simulink model "AR4FullPositionControl"  (R2026a)
settings: Solver=FixedStepAuto  StopTime=inf  FixedStep=3e-5
PreLoadFcn:
  | load('last_pos.mat');
StopFcn:
  | save('last_pos.mat', 'posJ6', 'posJ5', 'posJ4', 'posJ3', 'posJ2', 'posJ1', 'lastX', 'lastY', 'lastZ');
undefined symbols (not defined in the file): targetColor, targetGo, targetX, targetY, targetZ
libraries: arduinolib x31
(part 3 of 3)

== matlab function AR4FullPositionControl/Subsystem/J1/MATLAB Function1 ==
  data: startNext input; clk input; count output; dt input; rst input; displaySpeed output; dir output; pul output; next output; speedRPM input; positionAngle input; currCount input; accelRPMperSec input; limit output; mode input; homed output
function [count, displaySpeed, dir, pul, next, limit, homed] = J1(startNext, clk, dt, rst, speedRPM, positionAngle, currCount, accelRPMperSec, mode)
% J1 - Joint 1 position/speed controller with S-curve acceleration + HOMING
%
% AR4-MK3 robot. SINGLE-LIMIT joint.
% Limit switch at the most-positive end (+170 deg) = count 0.
% Count increases as the joint moves AWAY from the switch.
%
% MODE (single input):
%   mode = 0  ->  POSITION  : normal operation, drive to positionAngle input
%   mode = 1  ->  INITIALIZE: drive to HOME_TARGET, ignore positionAngle
%   mode = 2  ->  HOMING    : drive toward limit switch, zero count on contact
%
% Typical sequence: 2 (home) -> 1 (go to home angle) -> 0 (position control)
%
% INPUTS
%   startNext, clk, dt, rst, t, speedRPM, positionAngle, currCount,
%   accelRPMperSec, mode  (mode: 0=position, 1=initialize, 2=homing)
% OUTPUTS
%   count, displaySpeed, dir, pul, next, limit, homed
%
%   >>> J1: countsPerDeg=108.78  span=340 deg (-170..170)  maxCount=37500

    persistent currentCount lastClkState lastCount spTimer smoothedSpeed ...
               currentRPM distTraveled totalMoveFrozen lastTarget pulseAccum ...
               homedFlag lastMode;
    persistent chatterAccum chatterDir isStationary;

    % -------------------------------------------------------------------------
    % CONSTANTS  -  per-joint values
    % -------------------------------------------------------------------------
    Ts           = 3e-5;
    PPR          = 1000;
    CPR          = PPR * 4;
    maxCount     = 37500;          % <<< J1
    LIMIT_BUFFER = 50;
    TUNE_C2R     = 0.8;            % <<< J1

    TOTAL_DEG      = 340;          % <<< J1 span: 170-(-170)
    COUNTS_PER_REV = maxCount / TOTAL_DEG * 360;
    GEAR_RATIO     = COUNTS_PER_REV / CPR;
    C2R            = (GEAR_RATIO * CPR) / 60 * TUNE_C2R;

    speedUpdateInterval = 0.2;
    ALPHA               = 0.3;
    MIN_RPM             = 0.5;
    STOP_COUNTS         = 1;

    HOME_RPM    = 3;               % <<< tune: homing speed (RPM)
    HOME_TARGET = 90;               % <<< angle commanded in mode=1 (deg)

    % Single-limit angle->count mapping (anchored at switch)
    J_MIN_DEG    = -170;           % <<< J1
    J_MAX_DEG    =  170;           % <<< J1
    SWITCH_DEG   =  170;           % <<< J1 switch at +170 deg = count 0
    countsPerDeg = maxCount / TOTAL_DEG;

    % -------------------------------------------------------------------------
    % INITIALISATION (first call only)
    % -------------------------------------------------------------------------
    if isempty(currentCount)
        currentCount    = currCount;
        lastCount       = currCount;
        lastClkState    = clk;
        spTimer         = 0;
        smoothedSpeed   = 0;
        currentRPM      = MIN_RPM;
        distTraveled    = 0;
        totalMoveFrozen = 0;
        lastTarget      = -1;
        pulseAccum      = 0;
        homedFlag       = false;
        lastMode        = 0;
        chatterAccum    = 0;
        chatterDir      = 0;
        isStationary    = false;
    end

    limit = false;
    homed = homedFlag;
    dir   = 0;
    pul   = 0;
    next  = false;

    % -------------------------------------------------------------------------
    % 1. ENCODER COUNTING  (stop-triggered freeze)
    %
    % When the joint is stationary (last cycle's absError <= STOP_COUNTS),
    % ALL encoder edges are ignored -- the joint isn't supposed to be moving,
    % so any edge in that state is noise (encoder disk resting on a segment
    % boundary), not real motion. This is a hard freeze, not a filtered
    % accept: no edge can ever nudge currentCount while stationary, which
    % means no per-stop drift, and therefore no drift accumulation across
    % repeated stop events either.
    %
    % The moment a new target actually asks the joint to move (absError
    % grows past STOP_COUNTS, isStationary goes false), counting resumes
    % immediately and every edge is applied normally -- no debounce lag on
    % real motion.
    % -------------------------------------------------------------------------
    if clk ~= lastClkState && clk == 1
        if dt ~= clk
            edgeDir = 1;
        else
            edgeDir = -1;
        end

        if isStationary
            % FULL FREEZE while stationary. Any edge here is, by definition,
            % noise (the joint isn't supposed to be moving), so it's ignored
            % outright rather than "maybe accepted" -- this is what prevents
            % drift from accumulating across repeated stop events. Real
            % counting resumes automatically the moment isStationary goes
            % false (a new target actually asks the joint to move).
            chatterAccum = 0;
            chatterDir   = 0;
        else
            currentCount = currentCount + edgeDir;
            chatterAccum = 0;
            chatterDir   = 0;
        end
    end

    % Reset S-curve state on any mode change (once, on the transition)
    if mode ~= lastMode
        distTraveled    = 0;
        totalMoveFrozen = 0;
        pulseAccum      = 0;
        lastTarget      = -1;
        currentRPM      = MIN_RPM;
        spTimer         = 0;
        smoothedSpeed   = 0;
        chatterAccum    = 0;
        chatterDir      = 0;
    end
    lastMode = mode;

    % =========================================================================
    % MODE 2: HOMING
    % =========================================================================
    if mode == 2
        if rst == 1
            currentCount = 0;
            homedFlag    = true;
        end
        homed = homedFlag;          % limit NOT asserted during homing

        if homedFlag
            currentCount = 0;
            pul          = 0;
            next         = true;
        elseif startNext
            dir        = 0;         % toward switch = decreasing count
            pulseAccum = pulseAccum + HOME_RPM * C2R * Ts;
            if pulseAccum >= 1.0
                pul        = 1;
                pulseAccum = pulseAccum - 1.0;
            end
        end

        count        = currentCount;
        displaySpeed = HOME_RPM;
        lastClkState = clk;
        isStationary = false;
        return;
    end
    % =========================================================================

    % -------------------------------------------------------------------------
    % 2. SPEED DISPLAY
    % -------------------------------------------------------------------------
    spTimer = spTimer + Ts;
    if spTimer >= speedUpdateInterval
        smoothedSpeed = ALPHA * currentRPM + (1 - ALPHA) * smoothedSpeed;
        spTimer       = 0;
    end

    % -------------------------------------------------------------------------
    % 3. TARGET FROM ANGLE
    %    mode 1 (INITIALIZE): command = HOME_TARGET
    %    mode 0 (POSITION)  : command = positionAngle input
    % -------------------------------------------------------------------------
    if mode == 1
        cmdAngle = HOME_TARGET;
    else
        cmdAngle = positionAngle;
    end

    % Clamp to physical range, then map (single-limit, anchored at switch)
    if cmdAngle < J_MIN_DEG, cmdAngle = J_MIN_DEG; end
    if cmdAngle > J_MAX_DEG, cmdAngle = J_MAX_DEG; end
    targetCount = round(abs(SWITCH_DEG - cmdAngle) * countsPerDeg);
    targetCount = max(LIMIT_BUFFER, min(maxCount - LIMIT_BUFFER, targetCount));

    % -------------------------------------------------------------------------
    % 4. DIRECTION
    % -------------------------------------------------------------------------
    countError = targetCount - currentCount;
    absError   = abs(countError);
    if countError >= 0
        dir = 1;
    else
        dir = 0;
    end

    % -------------------------------------------------------------------------
    % 5. FREEZE totalMove ON NEW TARGET
    % -------------------------------------------------------------------------
    if targetCount ~= lastTarget
        totalMoveFrozen = absError;
        distTraveled    = 0;
        pulseAccum      = 0;
        lastTarget      = targetCount;
    end

    % -------------------------------------------------------------------------
    % 6. S-CURVE SPEED PROFILE
    % -------------------------------------------------------------------------
    accel = max(accelRPMperSec, 0.1);
    fullRampCounts = 0.5 * (MIN_RPM + speedRPM) * C2R * (speedRPM - MIN_RPM) / accel;

    if totalMoveFrozen > 0 && 2 * fullRampCounts >= totalMoveFrozen
        peakRPM    = sqrt(max(MIN_RPM^2 + totalMoveFrozen * accel / C2R, MIN_RPM^2));
        peakRPM    = max(MIN_RPM, min(speedRPM, peakRPM));
        rampCounts = 0.5 * (MIN_RPM + peakRPM) * C2R * (peakRPM - MIN_RPM) / accel;
        rampCounts = max(1, rampCounts);
    else
        peakRPM    = speedRPM;
        rampCounts = max(1, fullRampCounts);
    end

    if totalMoveFrozen <= 0
        targetRPM = MIN_RPM;
    elseif absError <= rampCounts
        x         = max(0.0, min(1.0, absError / rampCounts));
        targetRPM = MIN_RPM + (peakRPM - MIN_RPM) * 0.5 * (1 - cos(pi * x));
    elseif distTraveled <= rampCounts
        x         = max(0.0, min(1.0, distTraveled / rampCounts));
        targetRPM = MIN_RPM + (peakRPM - MIN_RPM) * 0.5 * (1 - cos(pi * x));
    else
        targetRPM = peakRPM;
    end
    currentRPM = max(MIN_RPM, min(speedRPM, targetRPM));

    % -------------------------------------------------------------------------
    % 7. DDS PULSE ACCUMULATOR
    % -------------------------------------------------------------------------
    if startNext && absError > STOP_COUNTS
        pulseAccum = pulseAccum + currentRPM * C2R * Ts;
        if pulseAccum >= 1.0
            pul          = 1;
            pulseAccum   = pulseAccum - 1.0;
            distTraveled = distTraveled + 1;
        end
        next = false;
    else
        next       = (absError <= STOP_COUNTS);
        pulseAccum = 0;
    end

    % -------------------------------------------------------------------------
    % 8. LIMIT SWITCH SAFETY (modes 0 and 1 only)
    % -------------------------------------------------------------------------
    if homedFlag && currentCount > LIMIT_BUFFER
        homedFlag = false;
    end
    if rst == 1 && ~homedFlag && dir == 0
        limit = true;
        pul   = 0;
    end
    if currentCount > maxCount
        limit = true;
        pul   = 0;
    end

    % -------------------------------------------------------------------------
    % 8.5 MODE-0 PULSE SUPPRESSION
    %     In position mode, CoordMove owns all pulse/dir generation.
    %     Force this block's own pul/dir to 0 so it can't leak a second
    %     pulse stream to the driver. Encoder counting + limit safety above
    %     still run normally every tick.
    % -------------------------------------------------------------------------
    if mode == 0
        pul = 0;
    end

    % -------------------------------------------------------------------------
    % 9. OUTPUTS
    % -------------------------------------------------------------------------
    count        = currentCount;
    displaySpeed = smoothedSpeed;
    homed        = homedFlag;
    lastClkState = clk;

    isStationary = (absError <= STOP_COUNTS);

end

== matlab function AR4FullPositionControl/MATLAB Function ==
  data: px input; J1 output; py input; pz input; J2 output; J3 output; J4 output; J5 output; J6 output
function [J1, J2, J3, J4, J5, J6] = AR4_IK(px, py, pz)
%AR4_IK  Analytical inverse kinematics for the AR4 MK3 6-axis robot arm.
%
%   [J1,J2,J3,J4,J5,J6] = AR4_IK(px, py, pz)
%
%   INPUTS
%     px, py, pz  – TCP position in mm
%
%   OUTPUTS
%     J1 … J6  – Joint command angles in DEGREES
%                (zero = mechanical home, matches AR4 software convention)
%
%   ORIENTATION
%     Hardcoded for top-down pick & place:
%       Rz = 180°, Ry = 0°, Rx = 180°  (gripper pointing straight down)
%     Change Rz_deg / Ry_deg / Rx_deg below if a different tool orientation
%     is needed.
%
%   DH PARAMETERS  (standard DH, from AR4 MK3 spreadsheet)
%     Joint | alpha      | d (mm)  | a (mm)
%     ------+------------+---------+-------
%       1   | -pi/2      | 169.77  |  64.2
%       2   |  0         |   0     | 305.0
%       3   |  pi/2      |   0     |   0
%       4   | -pi/2      | 222.63  |   0
%       5   |  pi/2      |   0     |   0
%       6   |  0         |  41.0   |   0
%
%   DH THETA OFFSETS  (DH_theta = cmd_angle_deg + offset_deg)
%     J1:  0°   J2: -90°   J3: 180°   J4: 0°   J5: 0°   J6: 0°
%
%     NOTE on J5: the offset is 0°, NOT +90°. This matches the AR4
%     software output. At mechanical home (J5_cmd = 90°), DH_theta = 90°.
%
%   JOINT LIMITS (command degrees)
%     J1 ±170   J2 -42/+90   J3 -89/+52
%     J4 ±165   J5 ±105      J6 ±155

% ── Link parameters ──────────────────────────────────────────────────────
a1 = 64.2;
d1 = 169.77;
a2 = 305.0;
d4 = 222.63;
d6 = 41.0;

% ── Tool orientation (change here if needed) ─────────────────────────────
Rz_deg = 180;
Ry_deg = 0;
Rx_deg = 180;
elbow_up = true;   % true = elbow-up (normal AR4 posture)

% ── Build R0_6 from ZYX extrinsic Euler angles ───────────────────────────
rz = Rz_deg * (pi/180);
ry = Ry_deg * (pi/180);
rx = Rx_deg * (pi/180);

Crz = cos(rz);  Srz = sin(rz);
Cry = cos(ry);  Sry = sin(ry);
Crx = cos(rx);  Srx = sin(rx);

R06 = [Crz*Cry,  Crz*Sry*Srx - Srz*Crx,  Crz*Sry*Crx + Srz*Srx; ...
       Srz*Cry,  Srz*Sry*Srx + Crz*Crx,  Srz*Sry*Crx - Crz*Srx; ...
      -Sry,      Cry*Srx,                 Cry*Crx               ];

% ── Wrist centre ─────────────────────────────────────────────────────────
% Pw = P_tcp - d6 * z_tool   (z_tool = 3rd column of R0_6)
approach = R06(:, 3);
Pw = [px; py; pz] - d6 * approach;
Wx = Pw(1);  Wy = Pw(2);  Wz = Pw(3);

% ── Joint 1 ──────────────────────────────────────────────────────────────
J1_rad = atan2(Wy, Wx);   % DH offset for J1 = 0

% ── Joints 2 & 3 (planar arm solution) ───────────────────────────────────
r = sqrt(Wx^2 + Wy^2) - a1;   % horizontal reach beyond J1 offset
s = Wz - d1;                   % vertical height above J2 axis

D = (r^2 + s^2 - a2^2 - d4^2) / (2 * a2 * d4);
D = max(-1.0, min(1.0, D));    % clamp numerical noise to [-1,1]

if elbow_up
    J3_raw = atan2(-sqrt(1 - D^2),  D);   % elbow-up: negative sqrt
else
    J3_raw = atan2( sqrt(1 - D^2),  D);   % elbow-down
end

J2_raw = atan2(s, r) - atan2(d4 * sin(J3_raw), a2 + d4 * cos(J3_raw));

% Convert geometric angles → command angles (remove DH theta offsets):
%   J2: DH offset = -pi/2  →  cmd = pi/2 - J2_raw
%   J3: DH offset =  pi    →  cmd = -J3_raw - pi/2
J2_rad = pi/2 - J2_raw;
J3_rad = -J3_raw - pi/2;

% ── Joints 4, 5, 6 (spherical wrist) ─────────────────────────────────────
R03 = dh_R03(J1_rad, J2_rad, J3_rad, a1, d1, a2);

R36 = R03' * R06;

% ZYZ-like wrist decomposition from R3_6:
J5_raw = atan2(sqrt(R36(1,3)^2 + R36(2,3)^2), R36(3,3));

if abs(sin(J5_raw)) > 1e-6
    J4_rad = atan2( R36(2,3) / sin(J5_raw),  R36(1,3) / sin(J5_raw));
    J6_rad = atan2( R36(3,2) / sin(J5_raw), -R36(3,1) / sin(J5_raw));
else
    % Gimbal lock (J5 ≈ 0° or 180°): absorb singularity into J4 = 0
    J4_rad = 0;
    if R36(3,3) > 0
        J6_rad = atan2(-R36(2,1),  R36(1,1));
    else
        J6_rad = atan2( R36(2,1), -R36(1,1));
    end
end

% J5 DH theta offset = 0  →  cmd = raw  (matches AR4 software)
J5_rad = J5_raw;

% ── Convert to degrees ────────────────────────────────────────────────────
J1 = J1_rad * (180/pi);
J2 = J2_rad * (180/pi);
J3 = J3_rad * (180/pi);
J4 = J4_rad * (180/pi);
J5 = J5_rad * (180/pi);
J6 = J6_rad * (180/pi);

end  % AR4_IK


% =========================================================================
%  Helper: rotation matrix R0_3  (joints 1-3 only)
% =========================================================================
function R03 = dh_R03(q1, q2, q3, a1, d1, a2)
%DH_R03  3×3 rotation submatrix of T0_3.
%  q1,q2,q3 are COMMAND angles in radians.

% DH theta offsets for joints 1-3
off = [0, -pi/2, pi];

% alpha for joints 1-3
al = [-pi/2, 0, pi/2];

% d for joints 1-3
dv = [d1, 0, 0];

% a for joints 1-3
av = [a1, a2, 0];

T = eye(4);
qs = [q1, q2, q3];

for i = 1:3
    th = qs(i) + off(i);
    ct = cos(th);  st = sin(th);
    ca = cos(al(i));  sa = sin(al(i));
    Ai = [ct, -st*ca,  st*sa, av(i)*ct; ...
          st,  ct*ca, -ct*sa, av(i)*st; ...
           0,     sa,     ca,     dv(i); ...
           0,      0,      0,        1];
    T = T * Ai;
end

R03 = T(1:3, 1:3);
end

== matlab function AR4FullPositionControl/Subsystem/J2/MATLAB Function1 ==
  data: startNext input; clk input; count output; dt input; rst input; displaySpeed output; dir output; pul output; next output; speedRPM input; positionAngle input; currCount input; accelRPMperSec input; limit output; mode input; homed output
function [count, displaySpeed, dir, pul, next, limit, homed] = J2(startNext, clk, dt, rst, speedRPM, positionAngle, currCount, accelRPMperSec, mode)
% J2 - Joint 2 position/speed controller with S-curve acceleration + HOMING
%
% AR4-MK3 robot. SINGLE-LIMIT joint.
% Limit switch at the most-negative end (-42 deg) = count 0.
% Count increases as the joint moves AWAY from the switch.
%
% MODE (single input):
%   mode = 0  ->  POSITION  : normal operation, drive to positionAngle input
%   mode = 1  ->  INITIALIZE: drive to HOME_TARGET, ignore positionAngle
%   mode = 2  ->  HOMING    : drive toward limit switch, zero count on contact
%
% Typical sequence: 2 (home) -> 1 (go to home angle) -> 0 (position control)
%
% INPUTS
%   startNext, clk, dt, rst, t, speedRPM, positionAngle, currCount,
%   accelRPMperSec, mode  (mode: 0=position, 1=initialize, 2=homing)
% OUTPUTS
%   count, displaySpeed, dir, pul, next, limit, homed
%
%   >>> J2: span=132 deg (-42..90)  maxCount=18300

    persistent currentCount lastClkState lastCount spTimer smoothedSpeed ...
               currentRPM distTraveled totalMoveFrozen lastTarget pulseAccum ...
               homedFlag lastMode;

    % -------------------------------------------------------------------------
    % CONSTANTS  -  per-joint values
    % -------------------------------------------------------------------------
    Ts           = 3e-5;
    PPR          = 1000;
    CPR          = PPR * 4;
    maxCount     = 18300;          % <<< J2
    LIMIT_BUFFER = 50;
    TUNE_C2R     = 0.8;            % <<< J2

    TOTAL_DEG      = 132;          % <<< J2 span: 90-(-42)
    COUNTS_PER_REV = maxCount / TOTAL_DEG * 360;
    GEAR_RATIO     = COUNTS_PER_REV / CPR;
    C2R            = (GEAR_RATIO * CPR) / 60 * TUNE_C2R;

    speedUpdateInterval = 0.2;
    ALPHA               = 0.3;
    MIN_RPM             = 0.5;
    STOP_COUNTS         = 1;

    HOME_RPM    = 2;               % <<< tune: homing speed (RPM)
    HOME_TARGET = 0;               % <<< angle commanded in mode=1 (deg)

    % Single-limit angle->count mapping (anchored at switch)
    J_MIN_DEG    = -42;            % <<< J2
    J_MAX_DEG    =  90;            % <<< J2
    SWITCH_DEG   = -42;            % <<< J2 switch at -42 deg = count 0
    countsPerDeg = maxCount / TOTAL_DEG;

    % -------------------------------------------------------------------------
    % INITIALISATION (first call only)
    % -------------------------------------------------------------------------
    if isempty(currentCount)
        currentCount    = currCount;
        lastCount       = currCount;
        lastClkState    = clk;
        spTimer         = 0;
        smoothedSpeed   = 0;
        currentRPM      = MIN_RPM;
        distTraveled    = 0;
        totalMoveFrozen = 0;
        lastTarget      = -1;
        pulseAccum      = 0;
        homedFlag       = false;
        lastMode        = 0;
    end

    limit = false;
    homed = homedFlag;
    dir   = 0;
    pul   = 0;
    next  = false;

    % -------------------------------------------------------------------------
    % 1. ENCODER COUNTING
    % -------------------------------------------------------------------------
    if clk ~= lastClkState && clk == 1
        if dt ~= clk
            currentCount = currentCount - 1;
        else
            currentCount = currentCount + 1;
        end
    end

    % Reset S-curve state on any mode change (once, on the transition)
    if mode ~= lastMode
        distTraveled    = 0;
        totalMoveFrozen = 0;
        pulseAccum      = 0;
        lastTarget      = -1;
        currentRPM      = MIN_RPM;
        spTimer         = 0;
        smoothedSpeed   = 0;
    end
    lastMode = mode;

    % =========================================================================
    % MODE 2: HOMING
    % =========================================================================
    if mode == 2
        if rst == 1
            currentCount = -235;
            homedFlag    = true;
        end
        homed = homedFlag;          % limit NOT asserted during homing

        if homedFlag
            currentCount = -235;
            pul          = 0;
            next         = true;
        elseif startNext
            dir        = 0;         % toward switch = decreasing count
            pulseAccum = pulseAccum + HOME_RPM * C2R * Ts;
            if pulseAccum >= 1.0
                pul        = 1;
                pulseAccum = pulseAccum - 1.0;
            end
        end

        count        = currentCount;
        displaySpeed = HOME_RPM;
        lastClkState = clk;
        return;
    end
    % =========================================================================

    % -------------------------------------------------------------------------
    % 2. SPEED DISPLAY
    % -------------------------------------------------------------------------
    spTimer = spTimer + Ts;
    if spTimer >= speedUpdateInterval
        smoothedSpeed = ALPHA * currentRPM + (1 - ALPHA) * smoothedSpeed;
        spTimer       = 0;
    end

    % -------------------------------------------------------------------------
    % 3. TARGET FROM ANGLE
    %    mode 1 (INITIALIZE): command = HOME_TARGET
    %    mode 0 (POSITION)  : command = positionAngle input
    % -------------------------------------------------------------------------
    if mode == 1
        cmdAngle = HOME_TARGET;
    else
        cmdAngle = positionAngle;
    end

    % Clamp to physical range, then map (single-limit, anchored at switch)
    if cmdAngle < J_MIN_DEG, cmdAngle = J_MIN_DEG; end
    if cmdAngle > J_MAX_DEG, cmdAngle = J_MAX_DEG; end
    targetCount = round(abs(SWITCH_DEG - cmdAngle) * countsPerDeg);
    targetCount = max(LIMIT_BUFFER, min(maxCount - LIMIT_BUFFER, targetCount));

    % -------------------------------------------------------------------------
    % 4. DIRECTION
    % -------------------------------------------------------------------------
    countError = targetCount - currentCount;
    absError   = abs(countError);
    if countError >= 0
        dir = 1;
    else
        dir = 0;
    end

    % -------------------------------------------------------------------------
    % 5. FREEZE totalMove ON NEW TARGET
    % -------------------------------------------------------------------------
    if targetCount ~= lastTarget
        totalMoveFrozen = absError;
        distTraveled    = 0;
        pulseAccum      = 0;
        lastTarget      = targetCount;
    end

    % -------------------------------------------------------------------------
    % 6. S-CURVE SPEED PROFILE
    % -------------------------------------------------------------------------
    accel = max(accelRPMperSec, 0.1);
    fullRampCounts = 0.5 * (MIN_RPM + speedRPM) * C2R * (speedRPM - MIN_RPM) / accel;

    if totalMoveFrozen > 0 && 2 * fullRampCounts >= totalMoveFrozen
        peakRPM    = sqrt(max(MIN_RPM^2 + totalMoveFrozen * accel / C2R, MIN_RPM^2));
        peakRPM    = max(MIN_RPM, min(speedRPM, peakRPM));
        rampCounts = 0.5 * (MIN_RPM + peakRPM) * C2R * (peakRPM - MIN_RPM) / accel;
        rampCounts = max(1, rampCounts);
    else
        peakRPM    = speedRPM;
        rampCounts = max(1, fullRampCounts);
    end

    if totalMoveFrozen <= 0
        targetRPM = MIN_RPM;
    elseif absError <= rampCounts
        x         = max(0.0, min(1.0, absError / rampCounts));
        targetRPM = MIN_RPM + (peakRPM - MIN_RPM) * 0.5 * (1 - cos(pi * x));
    elseif distTraveled <= rampCounts
        x         = max(0.0, min(1.0, distTraveled / rampCounts));
        targetRPM = MIN_RPM + (peakRPM - MIN_RPM) * 0.5 * (1 - cos(pi * x));
    else
        targetRPM = peakRPM;
    end
    currentRPM = max(MIN_RPM, min(speedRPM, targetRPM));

    % -------------------------------------------------------------------------
    % 7. DDS PULSE ACCUMULATOR
    % -------------------------------------------------------------------------
    if startNext && absError > STOP_COUNTS
        pulseAccum = pulseAccum + currentRPM * C2R * Ts;
        if pulseAccum >= 1.0
            pul          = 1;
            pulseAccum   = pulseAccum - 1.0;
            distTraveled = distTraveled + 1;
        end
        next = false;
    else
        next       = (absError <= STOP_COUNTS);
        pulseAccum = 0;
    end

    % -------------------------------------------------------------------------
    % 8. LIMIT SWITCH SAFETY (modes 0 and 1 only)
    % -------------------------------------------------------------------------
    if homedFlag && currentCount > LIMIT_BUFFER
        homedFlag = false;
    end
    if rst == 1 && ~homedFlag && dir == 0
        limit = true;
        pul   = 0;
    end
    if currentCount > maxCount
        limit = true;
        pul   = 0;
    end

    % -------------------------------------------------------------------------
    % 8.5 MODE-0 PULSE SUPPRESSION
    %     In position mode, CoordMove owns all pulse/dir generation.
    %     Force this block's own pul/dir to 0 so it can't leak a second
    %     pulse stream to the driver. Encoder counting + limit safety above
    %     still run normally every tick.
    % -------------------------------------------------------------------------
    if mode == 0
        pul = 0;
    end


    % -------------------------------------------------------------------------
    % 9. OUTPUTS
    % -------------------------------------------------------------------------
    count        = currentCount;
    displaySpeed = smoothedSpeed;
    homed        = homedFlag;
    lastClkState = clk;

end

== matlab function AR4FullPositionControl/Subsystem/J3/MATLAB Function1 ==
  data: startNext input; clk input; count output; dt input; rst input; displaySpeed output; dir output; pul output; next output; speedRPM input; positionAngle input; currCount input; accelRPMperSec input; limit output; mode input; homed output
function [count, displaySpeed, dir, pul, next, limit, homed] = J3(startNext, clk, dt, rst, speedRPM, positionAngle, currCount, accelRPMperSec, mode)
% J3 - Joint 3 position/speed controller with S-curve acceleration + HOMING
%
% AR4-MK3 robot. SINGLE-LIMIT joint.
% Limit switch at the most-positive end (+52 deg) = count 0.
% Count increases as the joint moves AWAY from the switch.
%
% MODE (single input):
%   mode = 0  ->  POSITION  : normal operation, drive to positionAngle input
%   mode = 1  ->  INITIALIZE: drive to HOME_TARGET, ignore positionAngle
%   mode = 2  ->  HOMING    : drive toward limit switch, zero count on contact
%
% Typical sequence: 2 (home) -> 1 (go to home angle) -> 0 (position control)
%
% INPUTS
%   startNext, clk, dt, rst, t, speedRPM, positionAngle, currCount,
%   accelRPMperSec, mode  (mode: 0=position, 1=initialize, 2=homing)
% OUTPUTS
%   count, displaySpeed, dir, pul, next, limit, homed
%
%   >>> J3: span=141 deg (-89..52)  maxCount=19720

    persistent currentCount lastClkState lastCount spTimer smoothedSpeed ...
               currentRPM distTraveled totalMoveFrozen lastTarget pulseAccum ...
               homedFlag lastMode;

    % -------------------------------------------------------------------------
    % CONSTANTS  -  per-joint values
    % -------------------------------------------------------------------------
    Ts           = 3e-5;
    PPR          = 1000;
    CPR          = PPR * 4;
    maxCount     = 19720;          % <<< J3
    LIMIT_BUFFER = 50;
    TUNE_C2R     = 0.8;            % <<< J3

    TOTAL_DEG      = 141;          % <<< J3 span: 52-(-89)
    COUNTS_PER_REV = maxCount / TOTAL_DEG * 360;
    GEAR_RATIO     = COUNTS_PER_REV / CPR;
    C2R            = (GEAR_RATIO * CPR) / 60 * TUNE_C2R;

    speedUpdateInterval = 0.2;
    ALPHA               = 0.3;
    MIN_RPM             = 0.5;
    STOP_COUNTS         = 1;

    HOME_RPM    = 3;               % <<< tune: homing speed (RPM)
    HOME_TARGET = 0;               % <<< angle commanded in mode=1 (deg)

    % Single-limit angle->count mapping (anchored at switch)
    J_MIN_DEG    = -89;            % <<< J3
    J_MAX_DEG    =  52;            % <<< J3
    SWITCH_DEG   =  52;            % <<< J3 switch at +52 deg = count 0
    countsPerDeg = maxCount / TOTAL_DEG;

    % -------------------------------------------------------------------------
    % INITIALISATION (first call only)
    % -------------------------------------------------------------------------
    if isempty(currentCount)
        currentCount    = currCount;
        lastCount       = currCount;
        lastClkState    = clk;
        spTimer         = 0;
        smoothedSpeed   = 0;
        currentRPM      = MIN_RPM;
        distTraveled    = 0;
        totalMoveFrozen = 0;
        lastTarget      = -1;
        pulseAccum      = 0;
        homedFlag       = false;
        lastMode        = 0;
    end

    limit = false;
    homed = homedFlag;
    dir   = 0;
    pul   = 0;
    next  = false;

    % -------------------------------------------------------------------------
    % 1. ENCODER COUNTING
    % -------------------------------------------------------------------------
    if clk ~= lastClkState && clk == 1
        if dt ~= clk
            currentCount = currentCount + 1;
        else
            currentCount = currentCount - 1;
        end
    end

    % Reset S-curve state on any mode change (once, on the transition)
    if mode ~= lastMode
        distTraveled    = 0;
        totalMoveFrozen = 0;
        pulseAccum      = 0;
        lastTarget      = -1;
        currentRPM      = MIN_RPM;
        spTimer         = 0;
        smoothedSpeed   = 0;
    end
    lastMode = mode;

    % =========================================================================
    % MODE 2: HOMING
    % =========================================================================
    if mode == 2
        if rst == 1
            currentCount = -1925;
            homedFlag    = true;
        end
        homed = homedFlag;          % limit NOT asserted during homing

        if homedFlag
            currentCount = -1925;
            pul          = 0;
            next         = true;
        elseif startNext
            dir        = 1;         % toward switch = decreasing count
            pulseAccum = pulseAccum + HOME_RPM * C2R * Ts;
            if pulseAccum >= 1.0
                pul        = 1;
                pulseAccum = pulseAccum - 1.0;
            end
        end

        count        = currentCount;
        displaySpeed = HOME_RPM;
        lastClkState = clk;
        return;
    end
    % =========================================================================

    % -------------------------------------------------------------------------
    % 2. SPEED DISPLAY
    % -------------------------------------------------------------------------
    spTimer = spTimer + Ts;
    if spTimer >= speedUpdateInterval
        smoothedSpeed = ALPHA * currentRPM + (1 - ALPHA) * smoothedSpeed;
        spTimer       = 0;
    end

    % -------------------------------------------------------------------------
    % 3. TARGET FROM ANGLE
    %    mode 1 (INITIALIZE): command = HOME_TARGET
    %    mode 0 (POSITION)  : command = positionAngle input
    % -------------------------------------------------------------------------
    if mode == 1
        cmdAngle = HOME_TARGET;
    else
        cmdAngle = positionAngle;
    end

    % Clamp to physical range, then map (single-limit, anchored at switch)
    if cmdAngle < J_MIN_DEG, cmdAngle = J_MIN_DEG; end
    if cmdAngle > J_MAX_DEG, cmdAngle = J_MAX_DEG; end
    targetCount = round(abs(SWITCH_DEG - cmdAngle) * countsPerDeg);
    targetCount = max(LIMIT_BUFFER, min(maxCount - LIMIT_BUFFER, targetCount));

    % -------------------------------------------------------------------------
    % 4. DIRECTION
    % -------------------------------------------------------------------------
    countError = targetCount - currentCount;
    absError   = abs(countError);
    if countError >= 0
        dir = 0;
    else
        dir = 1;
    end

    % -------------------------------------------------------------------------
    % 5. FREEZE totalMove ON NEW TARGET
    % -------------------------------------------------------------------------
    if targetCount ~= lastTarget
        totalMoveFrozen = absError;
        distTraveled    = 0;
        pulseAccum      = 0;
        lastTarget      = targetCount;
    end

    % -------------------------------------------------------------------------
    % 6. S-CURVE SPEED PROFILE
    % -------------------------------------------------------------------------
    accel = max(accelRPMperSec, 0.1);
    fullRampCounts = 0.5 * (MIN_RPM + speedRPM) * C2R * (speedRPM - MIN_RPM) / accel;

    if totalMoveFrozen > 0 && 2 * fullRampCounts >= totalMoveFrozen
        peakRPM    = sqrt(max(MIN_RPM^2 + totalMoveFrozen * accel / C2R, MIN_RPM^2));
        peakRPM    = max(MIN_RPM, min(speedRPM, peakRPM));
        rampCounts = 0.5 * (MIN_RPM + peakRPM) * C2R * (peakRPM - MIN_RPM) / accel;
        rampCounts = max(1, rampCounts);
    else
        peakRPM    = speedRPM;
        rampCounts = max(1, fullRampCounts);
    end

    if totalMoveFrozen <= 0
        targetRPM = MIN_RPM;
    elseif absError <= rampCounts
        x         = max(0.0, min(1.0, absError / rampCounts));
        targetRPM = MIN_RPM + (peakRPM - MIN_RPM) * 0.5 * (1 - cos(pi * x));
    elseif distTraveled <= rampCounts
        x         = max(0.0, min(1.0, distTraveled / rampCounts));
        targetRPM = MIN_RPM + (peakRPM - MIN_RPM) * 0.5 * (1 - cos(pi * x));
    else
        targetRPM = peakRPM;
    end
    currentRPM = max(MIN_RPM, min(speedRPM, targetRPM));

    % -------------------------------------------------------------------------
    % 7. DDS PULSE ACCUMULATOR
    % -------------------------------------------------------------------------
    if startNext && absError > STOP_COUNTS
        pulseAccum = pulseAccum + currentRPM * C2R * Ts;
        if pulseAccum >= 1.0
            pul          = 1;
            pulseAccum   = pulseAccum - 1.0;
            distTraveled = distTraveled + 1;
        end
        next = false;
    else
        next       = (absError <= STOP_COUNTS);
        pulseAccum = 0;
    end

    % -------------------------------------------------------------------------
    % 8. LIMIT SWITCH SAFETY (modes 0 and 1 only)
    % -------------------------------------------------------------------------
    if homedFlag && currentCount > LIMIT_BUFFER
        homedFlag = false;
    end
    if rst == 1 && ~homedFlag && dir == 1
        limit = true;
        pul   = 0;
    end
    if currentCount > maxCount
        limit = true;
        pul   = 0;
    end

    % -------------------------------------------------------------------------
    % 8.5 MODE-0 PULSE SUPPRESSION
    %     In position mode, CoordMove owns all pulse/dir generation.
    %     Force this block's own pul/dir to 0 so it can't leak a second
    %     pulse stream to the driver. Encoder counting + limit safety above
    %     still run normally every tick.
    % -------------------------------------------------------------------------
    if mode == 0
        pul = 0;
    end


    % -------------------------------------------------------------------------
    % 9. OUTPUTS
    % -------------------------------------------------------------------------
    count        = currentCount;
    displaySpeed = smoothedSpeed;
    homed        = homedFlag;
    lastClkState = clk;

end
